simulink model "susp_template"  (Simulink 6.3)
settings: Solver=ode45  StartTime=0.0  StopTime=4  RelTol=1e-6
values from neighbouring files (symbols this model uses):
  A = [0 1 0 0;-(kf/ms) -(ba/ms) (kf/ms) (ba/ms); 0 0 0 1; (kf/mr) (ba/mr) -(kf+kp)/mr -(ba/mr)]    [dados_susp.m]
  B = [0 0;0 -1/ms; 0 0;(kp/mr) (1/mr)]    [dados_susp.m]
  C = [1 0 0 0;0 1 0 0;0 0 1 0;0 0 0 1]    [dados_susp.m]
  Coff = 500    [dados_susp.m]
  Con = 1400    [dados_susp.m]
  D = [0 0; 0 0; 0 0; 0 0]    [dados_susp.m]
undefined symbols (not defined in the file or in its folder): susp_fuz
settings Model: LastModifiedBy=paiva  StrictBusMsg=None
settings DataIOCC: SignalLoggingName=sigsOut
settings DebuggingCC: SolverPrmCheckMsg=none
settings HardwareCC: TargetUnknown=on

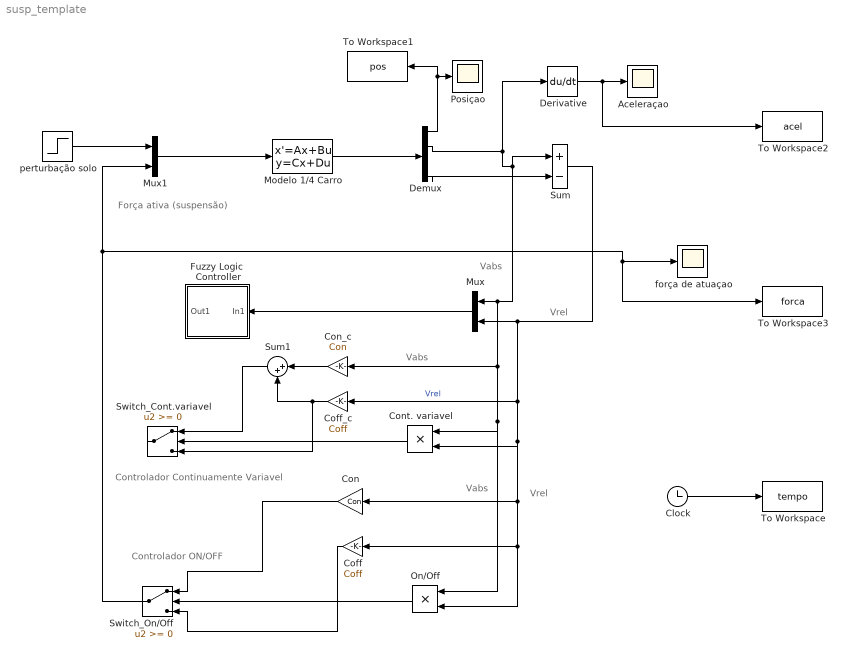
== system susp_template ==
  note: Vrel
  note: Vabs
  note: Vabs
  note: Vabs
  note: Vrel
  note: Força ativa (suspensão)
  note: Controlador
      | Continuamente Variavel
  note: Controlador ON/OFF
  Aceleraçao : Scope
      settings: TimeRange=2  YMin=-2  YMax=1  SaveName=Aceleraçao
  Clock : Clock
      settings: Decimation=10
  Coff : Gain  Orientation=left  Gain=Coff  SaturateOnIntegerOverflow=on
  Coff_c : Gain  Orientation=left  Gain=Coff  SaturateOnIntegerOverflow=on
  Con : Gain  Orientation=left  Gain=Con  SaturateOnIntegerOverflow=on
  Con_c : Gain  Orientation=left  Gain=Con  SaturateOnIntegerOverflow=on
  Cont. variavel : Product  Orientation=left  SaturateOnIntegerOverflow=on
  Demux : Demux
  Derivative : Derivative
  Fuzzy Logic  Controller : Subsystem  Orientation=left  AncestorBlock="fuzblock/Fuzzy Logic  Controller"  mask(FIS){fis=susp_fuz}
      mask prompts: fis "FIS File or Structure:"
      mask help: FIS
      mask init:
      | fis = fuzblockmask(gcb,fis);
      mask Help: web(['file:///' docroot '/toolbox/fuzzy/fuzzylogiccontroller.html']);
      mask Display: plot(0, -0.3, 6, -0.3, 0, 1.2, 6, 1.2, [0 6], [0 0], [1 2 3],[0 1 0],[2 3 4],[0 1 0],[3 4 5],[0 1 0])
  Modelo 1/4 Carro : StateSpace  A=A  B=B  C=C  D=D  X0=[0 0 0 0]
  Mux : Mux  Orientation=left  Inputs=2
  Mux1 : Mux  Inputs=2
  On/Off : Product  Orientation=left  SaturateOnIntegerOverflow=on
  Posiçao : Scope
      settings: TimeRange=2  YMin=-1.73472e-018  YMax=0.065  SaveName=posicao_chassis
  Sum : Sum  Inputs=|+-  SaturateOnIntegerOverflow=on
  Sum1 : Sum  Orientation=left  Inputs=|++  SaturateOnIntegerOverflow=on
  Switch_Cont.variavel : Switch  Orientation=left  SaturateOnIntegerOverflow=on
  Switch_On/Off : Switch  Orientation=left  SaturateOnIntegerOverflow=on
  To Workspace : ToWorkspace  VariableName=tempo  SampleTime=-1  SaveFormat=Array
  To Workspace1 : ToWorkspace  VariableName=pos  SampleTime=-1  SaveFormat=Array
  To Workspace2 : ToWorkspace  VariableName=acel  SampleTime=-1  SaveFormat=Array
  To Workspace3 : ToWorkspace  VariableName=forca  SampleTime=-1  SaveFormat=Array
  força de atuaçao : Scope
      settings: TimeRange=2  YMin=-2  YMax=1  SaveName=Aceleraao1
  perturbação solo : Step  Time=0  After=0.05  SampleTime=0  VectorParams1D=off  ZeroCross=off
  wires:
  Modelo 1/4 Carro/1 -> Demux/1
  Mux1/1 -> Modelo 1/4 Carro/1
  perturbação solo/1 -> Mux1/1
  Mux/1 -> Fuzzy Logic  Controller/1(In1)
  Demux/4 -> Sum/2
  Demux/2 -> Sum/1, Mux/1, Con_c/1, Cont. variavel/1, On/Off/1, Derivative/1
  Derivative/1 -> Aceleraçao/1, To Workspace2/1
  Demux/1 -> Posiçao/1, To Workspace1/1
  Sum/1 -> Mux/2, Coff_c/1, Cont. variavel/2, Con/1, On/Off/2, Coff/1  "Vrel"
  Cont. variavel/1 -> Switch_Cont.variavel/2
  Coff_c/1 -> Sum1/2, Switch_Cont.variavel/3
  Con_c/1 -> Sum1/1
  Sum1/1 -> Switch_Cont.variavel/1
  Clock/1 -> To Workspace/1
  On/Off/1 -> Switch_On/Off/2
  Con/1 -> Switch_On/Off/1
  Coff/1 -> Switch_On/Off/3
  Switch_On/Off/1 -> Mux1/2, força de atuaçao/1, To Workspace3/1

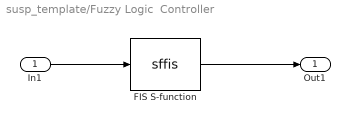
== system susp_template/Fuzzy Logic  Controller ==
  In1 : Inport
  FIS S-function : S-Function  FunctionName=sffis  Parameters=fis  SFunctionModules=sfsup
  Out1 : Outport
  wires:
  In1/1 -> FIS S-function/1
  FIS S-function/1 -> Out1/1
